simulink model "MODELODETURBINADERIOV9"  (R2018a)
settings: Solver=VariableStepAuto  StartTime=0.0  StopTime=0.5  FixedStep=50e-3  MaxStep=1e-4  RelTol=1e-3
undefined symbols (not defined in the file): A, B, beta, Ccc, Cinv, Dcc, den, Fr, J, K1Vo, K2Vo, Kb, Kp, Lcc, Linv, Lr, r, Rcc, Ri, Rinv, Rr, sigbuilder_block, T_d, Tc
libraries: powerlib x43, simulink x3, powerlib_meascontrol x1
settings Model: Creator=zni.uao  LastModifiedBy=cmparedes
settings SolverCC: ZeroCrossAlgorithm=Adaptive
settings OptimizationCC: LifeSpan=inf
settings DebuggingCC: SFExecutionAtInitializationDiag=none
settings HardwareCC: ProdBitPerPointer=32  ProdBitPerSizeT=32  ProdBitPerPtrDiffT=32  ProdLargestAtomicFloat=None  ProdWordSize=32  ProdHWDeviceType=Custom Processor->Custom
settings CodeAppCC: StateflowObjectComments=on
settings SimscapeCC: SimscapeNormalizeSystem=off

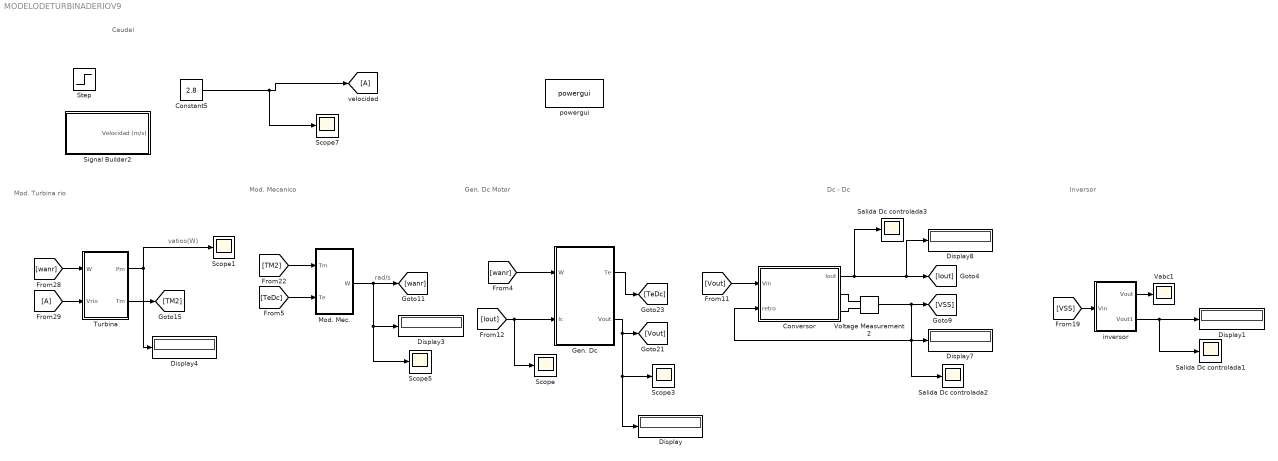
== system MODELODETURBINADERIOV9 ==
  note: rad/s
  note: Mod. Turbina rio
  note: Mod. Mecanico
  note: Caudal
  note: Gen. Dc Motor
  note: Dc - Dc
  note: Inversor
  note: vatios(W)
  Constant5 : Constant  Value=2.8
  Conversor : Subsystem
  Display{,1,3..4,7..8} (6 alike) : Display
  Gen. Dc : Subsystem
  Mod. Mec. : Subsystem
  Salida Dc controlada1 : Scope
  Salida Dc controlada2 : Scope
  Salida Dc controlada3 : Scope
  Scope{,1,3,5,7} (5 alike) : Scope
  Signal Builder2 : Subsystem  Tag=STV Subsys  LoadFcn=sigbuilder_block('load');  StartFcn=sigbuilder_block('start');  StopFcn=sigbuilder_block('stop');  ClipboardFcn=sigbuilder_block('clipboard');  mask(Sigbuilder block){tuvar=[0:10]}
      mask help: Simulink:masks:SigbuilderBlock_MD
      mask init:
      | if ~strcmp(get_param(bdroot(gcbh),'SimulationStatus'),'stopped') tuvar = sigbuilder_block('maskInit'); end
      settings: CopyFcn=sigbuilder_block('copy');  DeleteFcn=sigbuilder_block('delete');  ModelCloseFcn=sigbuilder_block('modelClose');  PreSaveFcn=sigbuilder_block('preSave');  PauseFcn=sigbuilder_block('pause');  ContinueFcn=sigbuilder_block('continue');  NameChangeFcn=sigbuilder_block('namechange');  OpenFcn=sigbuilder_block('open',[197.25 66 550.5 359.25 ]);  CloseFcn=sigbuilder_block('close');
      mask Display: plot(0, 0, 100, 100,[2, 2, 32, 32, 2], [68, 8, 8, 68, 68],[32, 2], [38, 38], [32, 19, 2],[53, 60, 44], [32, 17, 17, 2],[16, 16, 31, 31]);txt = getActiveGroup(gcbh);text(2, 100, txt,'verticalAlignment', 'top');
  Step : Step  Time=10  Before=2.5  After=2.888  SampleTime=0
  Turbina : Subsystem
  Vabc1 : Scope
  Voltage Measurement2 : powerlib/Measurements/Voltage Measurement  PhasorSimulation=off  OutputType=Complex  PSBequivalent=0
  inversor : Subsystem
  powergui : powerlib/powergui  Priority=1  SimulationMode=Continuous  SampleTime=50e-3  frequency=60  Iterations=50  frequencyindice=0  Pbase=100e6  ErrMax=1e-4  UnitsV=kV  UnitsW=MW  buscounter=0  FunctionMessages=off  echomessages=off  EnableUseOfTLC=off  CurrentSourceSwitches=off  DisableSnubberDevices=off  DisableRonSwitches=off  DisableVfSwitches=off  DisplayEquations=off  SolverType=Tustin/Backward Euler (TBE)  Interpol=off  ExternalGateDelay=off  methode=off  Ts=100  x0status=blocks  SPID=on  SwTol=0  HookPort=off  RestoreLinks=warning  ResistiveCurrentMeasurement=off  Frange=[0:2:500]  Ylog=off  Xlog=on  ShowGrid=off  save=off  variable=ZData  structure=0  ZoomFFT=off  StartTime=0.0  cycles=1  DisplayStyle=1  fundamental=60  FreqAxis=off  MaxFrequency=1000  frequencyindicesteady=0 Hz  RmsSteady=1  display=off
  wires:
  [wanr] -> Turbina/1(W)
  [A] -> Turbina/2(Vrio)
  Turbina/1(Pm) -> Scope1/1, Display4/1
  Turbina/2(Tm) -> [TM2]
  Mod. Mec./1(W) -> Display3/1, Scope5/1, [wanr]
  [TM2] -> Mod. Mec./1(Tm)
  Gen. Dc/1(Te) -> [TeDc]
  [TeDc] -> Mod. Mec./2(Te)
  Constant5/1 -> Scope7/1, [A]
  [wanr] -> Gen. Dc/1(W)
  [VSS] -> inversor/1(Vin)
  [Iout] -> Scope/1, Gen. Dc/2(Ic)
  Gen. Dc/2(Vout) -> [Vout], Scope3/1, Display/1
  Voltage Measurement2/1 -> [VSS], Conversor/2(retro), Salida Dc controlada2/1, Display7/1
  Conversor/1(Iout) -> Salida Dc controlada3/1, Display8/1, [Iout]
  inversor/1(Vout) -> Vabc1/1
  [Vout] -> Conversor/1(Vin)
  inversor/2(Vout1) -> Salida Dc controlada1/1, Display1/1
  connections:
  Voltage Measurement2/LConn1 -- Conversor/RConn1
  Voltage Measurement2/LConn2 -- Conversor/RConn2

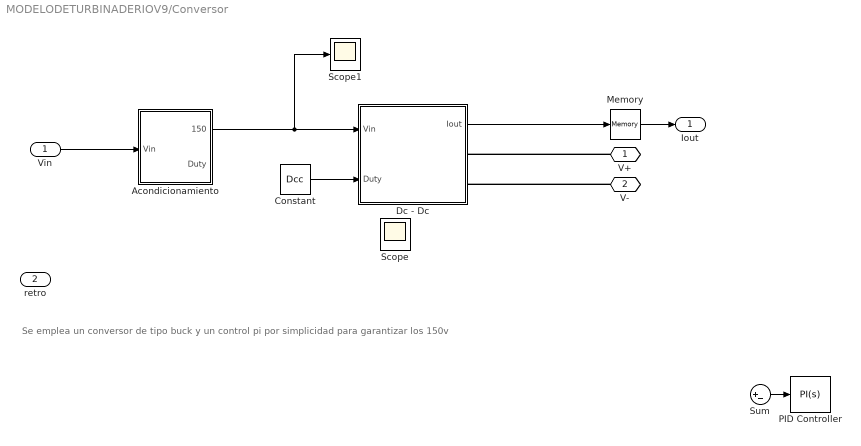
== system MODELODETURBINADERIOV9/Conversor ==
  note: Se emplea un conversor de tipo buck y un control pi por simplicidad para garantizar los 150v
  Vin : Inport
  retro : Inport  Port=2
  Acondicionamiento : Subsystem
  Constant : Constant  Value=Dcc
  Dc - Dc : Subsystem
  Memory : Memory
  PID Controller : simulink/Continuous/PID Controller  Controller=PI  TimeDomain=Continuous-time  SampleTime=-1  IntegratorMethod=Forward Euler  FilterMethod=Forward Euler  Form=Parallel  UseFilter=on  ControllerParametersSource=internal  P=0  I=49.9781304897077  D=1.18866706411967e-05  N=181963.738974805  InitialConditionSource=internal  InitialConditionForIntegrator=0  InitialConditionForFilter=0  ExternalReset=none  LimitOutput=off  UpperSaturationLimit=inf  LowerSaturationLimit=-inf  LinearizeAsGain=on  AntiWindupMode=none  Kb=1  TrackingMode=off  Kt=1  PParamMin=[]  PParamMax=[]  IParamMin=[]  IParamMax=[]  DParamMin=[]  DParamMax=[]  NParamMin=[]  NParamMax=[]  KbParamMin=[]  KbParamMax=[]  KtParamMin=[]  KtParamMax=[]  POutMin=[]  POutMax=[]  IOutMin=[]  IOutMax=[]  DOutMin=[]  DOutMax=[]  NOutMin=[]  NOutMax=[]  KbOutMin=[]  KbOutMax=[]  KtOutMin=[]  KtOutMax=[]  IntegratorOutMin=[]  IntegratorOutMax=[]  FilterOutMin=[]  FilterOutMax=[]  SumOutMin=[]  SumOutMax=[]  SumI1OutMin=[]  SumI1OutMax=[]  SumI2OutMin=[]  SumI2OutMax=[]  SumI3OutMin=[]  SumI3OutMax=[]  SumDOutMin=[]  SumDOutMax=[]  SaturationOutMin=[]  SaturationOutMax=[]  IntegratorContinuousStateAttributes=''  IntegratorStateMustResolveToSignalObject=off  IntegratorRTWStateStorageClass=Auto  FilterContinuousStateAttributes=''  FilterStateMustResolveToSignalObject=off  FilterRTWStateStorageClass=Auto  DifferentiatorICPrevScaledInput=0  DifferentiatorOutMin=[]  DifferentiatorOutMax=[]  InitialConditionSetting=State (most efficient)  FilterDiffOutCoefMin=[]  FilterDiffOutCoefMax=[]  SumDenOutMin=[]  SumDenOutMax=[]  SumNumOutMin=[]  SumNumOutMax=[]  ReciprocalOutMin=[]  ReciprocalOutMax=[]  DivideOutMin=[]  DivideOutMax=[]  TunerSelectOption=Transfer Function Based (PID Tuner App)
  Scope : Scope
  Scope1 : Scope
  Sum : Sum  Inputs=|+-
  V+ : PMIOPort  Side=Right
  V- : PMIOPort  Port=2  Side=Right
  Iout : Outport
  wires:
  Dc - Dc/1(Iout) -> Memory/1
  Acondicionamiento/1(150) -> Scope1/1, Dc - Dc/1(Vin)
  Memory/1 -> Iout/1
  Vin/1 -> Acondicionamiento/1(Vin)
  ? -> Sum/1
  Sum/1 -> PID Controller/1
  ? -> Sum/2
  Constant/1 -> Dc - Dc/2(Duty)
  connections:
  V+/RConn1 -- Dc - Dc/RConn1
  V-/RConn1 -- Dc - Dc/RConn2

== system MODELODETURBINADERIOV9/Gen. Dc ==
  note: Calculo del par electrico con la corriente en la carga
  note: Se emplean parametro de un motor dc para 18.5Kw debido a que fueron con los que mejor trabajo
  W : Inport
  Ic : Inport  Port=2
  Motor iman. : Subsystem
  Par elec. : Subsystem
  Te : Outport
  Vout : Outport  Port=2
  wires:
  Motor iman./1(Out1) -> Vout/1
  Par elec./1(Te) -> Te/1
  W/1 -> Motor iman./2(W)
  Ic/1 -> Par elec./1(Ic), Motor iman./1(I)

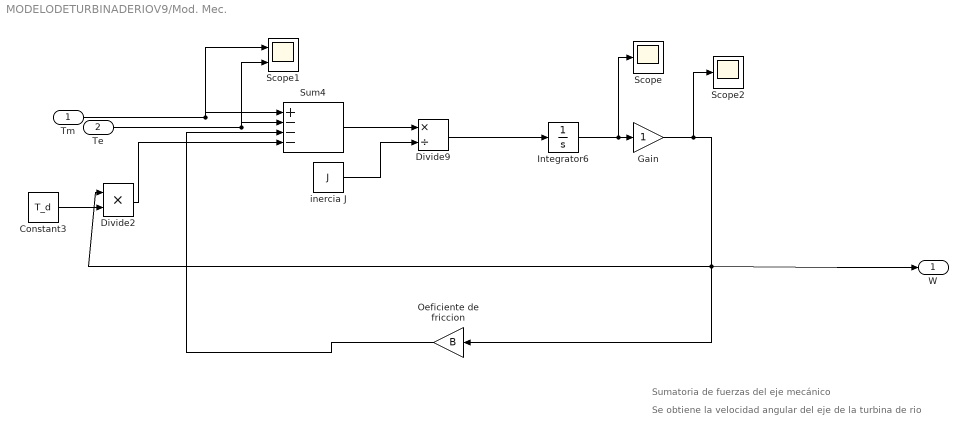
== system MODELODETURBINADERIOV9/Mod. Mec. ==
  note: Se obtiene la velocidad angular del eje de la turbina de rio
  note: Sumatoria de fuerzas del eje mecánico
  Tm : Inport
  Te : Inport  Port=2
  Constant3 : Constant  Value=T_d
  Divide2 : Product  Inputs=**
  Divide9 : Product  Inputs=*/
  Gain : Gain
  Integrator6 : Integrator  InitialCondition=10
  Oeficiente de friccion : Gain  Gain=B
  Scope : Scope
  Scope1 : Scope  NumInputPorts=2
  Scope2 : Scope
  Sum4 : Sum  Inputs=|+---
  inercia J : Constant  Value=J
  W : Outport
  wires:
  inercia J/1 -> Divide9/2
  Constant3/1 -> Divide2/2
  Divide2/1 -> Sum4/4
  Oeficiente de friccion/1 -> Sum4/3
  Sum4/1 -> Divide9/1
  Tm/1 -> Scope1/1, Sum4/1
  Te/1 -> Scope1/2, Sum4/2
  Divide9/1 -> Integrator6/1
  Integrator6/1 -> Scope/1, Gain/1
  Gain/1 -> Scope2/1, Oeficiente de friccion/1, W/1, Divide2/1

== system MODELODETURBINADERIOV9/Signal Builder2 ==
  Demux : Demux  Tag=STV Demux  Outputs=1
  FromWs : FromWorkspace  Tag=STV FromWs  VariableName=tuvar  SampleTime=0
      SigBuilderData=|
      | common.afterFinalStr = 'Extrapolate'
      | common.sampleTime = 0
      | dataSet.timeRange = [0 0.1]
      | dataSet.name = 'Group 1'
      | sbobj.Groups.Name = 'Group 1'
      | sbobj.Groups.Signals.Name = 'Velocidad (m/s)'
      | sbobj.Groups.Signals.XData = [0 0.01 0.01 0.02 0.02 0.0298 0.0298 0.0398 0.0498 0.06 0.1]
      | sbobj.Groups.Signals.YData = [2 2 2.5 2.5 2.595 2.595 2.8 2.8 2.8 2.8 2.8]
      | sbobj.Groups.TimeRange = [0 0.1]
  Velocidad (m/s) : Outport  Tag=STV Outport
  wires:
  FromWs/1 -> Demux/1
  Demux/1 -> Velocidad (m/s)/1

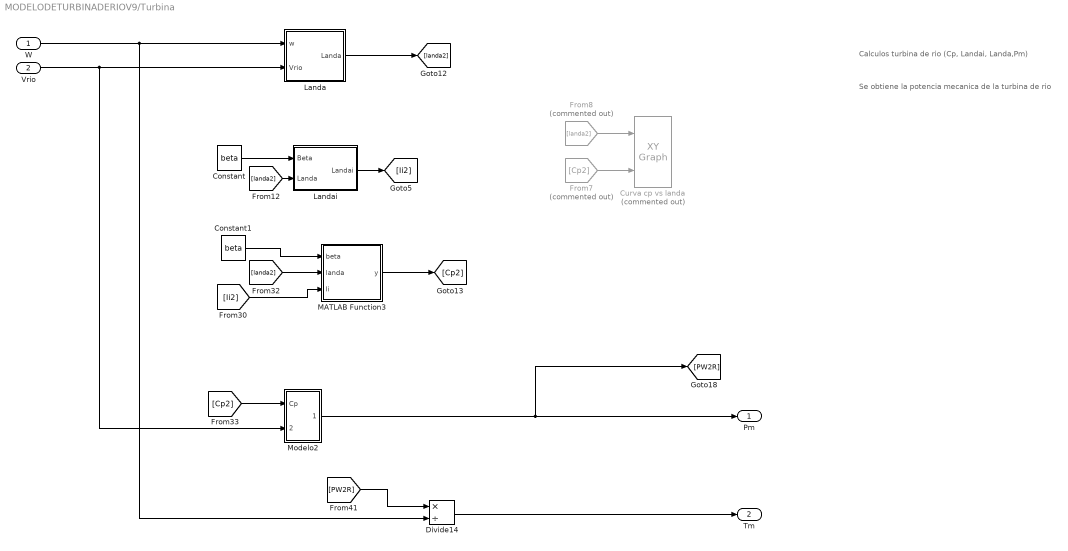
== system MODELODETURBINADERIOV9/Turbina ==
  note: Calculos turbina de rio (Cp, Landai, Landa,Pm)
  note: Se obtiene la potencia mecanica de la turbina de rio
  W : Inport
  Vrio : Inport  Port=2
  Constant : Constant  Value=beta
  Constant1 : Constant  Value=beta
  Curva cp vs landa : simulink/Sinks/XY Graph  Commented=on  xmin=1  xmax=20  ymin=0  ymax=0.56  st=0.1
  Divide14 : Product  Inputs=*/
  From7 : From  Commented=on  GotoTag=Cp2
  From8 : From  Commented=on  GotoTag=landa2
  Landa : Subsystem
  Landai : Subsystem
  MATLAB Function3 : MATLAB Function  TreatAsAtomicUnit=on
  Modelo2 : Subsystem
  Pm : Outport
  Tm : Outport  Port=2
  wires:
  Constant1/1 -> MATLAB Function3/1(beta)
  Divide14/1 -> Tm/1
  [Ii2] -> MATLAB Function3/3(Ii)
  [Cp2] -> Modelo2/1(Cp)
  [PW2R] -> Divide14/1
  W/1 -> Divide14/2, Landa/1(w)
  [landa2] -> MATLAB Function3/2(landa)
  Vrio/1 -> Modelo2/2(Vrio), Landa/2(Vrio)
  Landa/1(Landa) -> [landa2]
  MATLAB Function3/1(y) -> [Cp2]
  From8/1 -> Curva cp vs landa/1
  Constant/1 -> Landai/1(Beta)
  [landa2] -> Landai/2(Landa)
  Modelo2/1(Pm) -> [PW2R], Pm/1
  Landai/1(Landai) -> [Ii2]
  From7/1 -> Curva cp vs landa/2

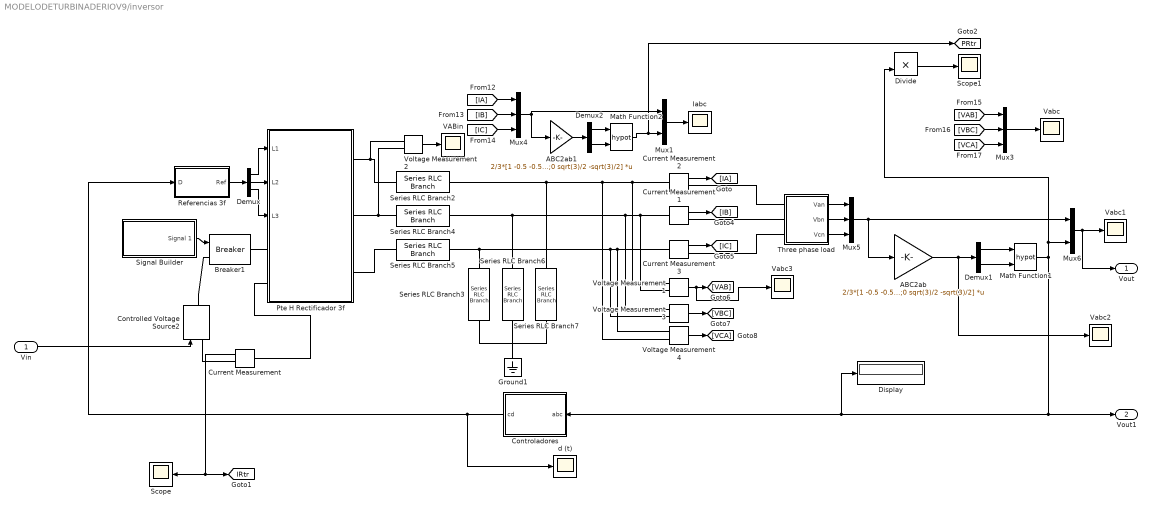
== system MODELODETURBINADERIOV9/inversor ==
  Vin : Inport
  ABC2ab : Gain  Gain=2/3*[1 -0.5 -0.5;0 sqrt(3)/2 -sqrt(3)/2]  Multiplication=Matrix(K*u)  SaturateOnIntegerOverflow=on  OutDataTypeStr=Inherit: Same as input  ParamDataTypeStr=Inherit: Same as input
  ABC2ab1 : Gain  Gain=2/3*[1 -0.5 -0.5;0 sqrt(3)/2 -sqrt(3)/2]  Multiplication=Matrix(K*u)  SaturateOnIntegerOverflow=on  OutDataTypeStr=Inherit: Same as input  ParamDataTypeStr=Inherit: Same as input
  Breaker1 : powerlib/Elements/Breaker  InitialState=0  SwitchingTimes="[ 1/60  5/60 ]"  External=on  BreakerResistance=0.01  SnubberResistance=1e6  SnubberCapacitance=inf  Measurements=None  MoreParameters=off  NoBreakLoop=off
      settings: SourceProductName=Simscape Power Systems
  Controladores : Subsystem
  Controlled Voltage Source2 : powerlib/Electrical Sources/Controlled Voltage Source  Initialize=on  Source_Type=DC  Amplitude=150  Phase=0  Frequency=0  Measurements=None
  Current Measurement{,1..3} (4 alike) : powerlib/Measurements/Current Measurement  PhasorSimulation=off  OutputType=Complex  PSBequivalent=0
  Demux : Demux  Outputs=3
  Demux1 : Demux  Outputs=2
  Demux2 : Demux  Outputs=2
  Display : Display
  Divide : Product  Inputs=**
  Ground1 : powerlib/Elements/Ground  LConnTagsString=a
  Iabc : Scope
  Math Function1 : Math  Operator=hypot  SaturateOnIntegerOverflow=on
  Math Function2 : Math  Operator=hypot  SaturateOnIntegerOverflow=on
  Mux1 : Mux  Inputs=2
  Mux3 : Mux  Inputs=3
  Mux4 : Mux  Inputs=3
  Mux5 : Mux  Inputs=3
  Mux6 : Mux  Inputs=2
  Pte H Rectificador 3f : Subsystem
  Referencias 3f : Subsystem
  Scope : Scope
  Scope1 : Scope
  Series RLC Branch2 : powerlib/Elements/Series RLC Branch  LConnTagsString=__new0  RConnTagsString=__new0  BranchType=RL  Resistance=Rinv  Inductance=Linv  SetiL0=off  InitialCurrent=0  Capacitance=1.0  Setx0=off  InitialVoltage=0  Measurements=None
  Series RLC Branch3 : powerlib/Elements/Series RLC Branch  LConnTagsString=__new0  RConnTagsString=__new0  BranchType=C  Resistance=0.01  Inductance=1e-3  SetiL0=off  InitialCurrent=0  Capacitance=Cinv  Setx0=on  InitialVoltage=311  Measurements=None
  Series RLC Branch4 : powerlib/Elements/Series RLC Branch  LConnTagsString=__new0  RConnTagsString=__new0  BranchType=RL  Resistance=Rinv  Inductance=Linv  SetiL0=off  InitialCurrent=0  Capacitance=1.0  Setx0=off  InitialVoltage=0  Measurements=None
  Series RLC Branch5 : powerlib/Elements/Series RLC Branch  LConnTagsString=__new0  RConnTagsString=__new0  BranchType=RL  Resistance=Rinv  Inductance=Linv  SetiL0=off  InitialCurrent=0  Capacitance=1.0  Setx0=off  InitialVoltage=0  Measurements=None
  Series RLC Branch6 : powerlib/Elements/Series RLC Branch  LConnTagsString=__new0  RConnTagsString=__new0  BranchType=C  Resistance=0.01  Inductance=1e-3  SetiL0=off  InitialCurrent=0  Capacitance=Cinv  Setx0=on  InitialVoltage=311  Measurements=None
  Series RLC Branch7 : powerlib/Elements/Series RLC Branch  LConnTagsString=__new0  RConnTagsString=__new0  BranchType=C  Resistance=0.01  Inductance=1e-3  SetiL0=off  InitialCurrent=0  Capacitance=Cinv  Setx0=on  InitialVoltage=311  Measurements=None
  Signal Builder : Subsystem  Tag=STV Subsys  LoadFcn=sigbuilder_block('load');  StartFcn=sigbuilder_block('start');  StopFcn=sigbuilder_block('stop');  ClipboardFcn=sigbuilder_block('clipboard');  mask(Sigbuilder block){tuvar=[0:10]}
      mask help: Sigbuilder GUI
      mask init:
      | if ~strcmp(get_param(bdroot(gcbh),'SimulationStatus'),'stopped') tuvar = sigbuilder_block('maskInit'); end
      settings: CopyFcn=sigbuilder_block('copy');  DeleteFcn=sigbuilder_block('delete');  ModelCloseFcn=sigbuilder_block('modelClose');  PreSaveFcn=sigbuilder_block('preSave');  PauseFcn=sigbuilder_block('pause')  ContinueFcn=sigbuilder_block('continue')  NameChangeFcn=sigbuilder_block('namechange');  OpenFcn=sigbuilder_block('open',[437.25 117 550.5 399 ]);  CloseFcn=sigbuilder_block('close');
      mask Display: plot(0, 0, 100, 100,[2, 2, 32, 32, 2], [68, 8, 8, 68, 68],[32, 2], [38, 38], [32, 19, 2],[53, 60, 44], [32, 17, 17, 2],[16, 16, 31, 31]);txt = getActiveGroup(gcbh);text(2, 100, txt,'verticalAlignment', 'top');
  Three phase load : Subsystem
  VABin : Scope
  Vabc{,1..3} (4 alike) : Scope
  Voltage Measurement{1..4} (4 alike) : powerlib/Measurements/Voltage Measurement  PhasorSimulation=off  OutputType=Complex  PSBequivalent=0
  d (t) : Scope
  Vout : Outport
  Vout1 : Outport  Port=2
  tag scope: IRtr=global, PRtr=global
  wires:
  Demux/3 -> Pte H Rectificador 3f/3(L3)
  Referencias 3f/1(Ref) -> Demux/1
  [VBC] -> Mux3/2
  Three phase load/3(Vcn) -> Mux5/3
  Three phase load/1(Van) -> Mux5/1
  ABC2ab1/1 -> Demux2/1
  Current Measurement3/1 -> [IC]
  Mux5/1 -> Mux6/1, ABC2ab/1
  Demux2/1 -> Math Function2/1
  [VCA] -> Mux3/3
  [IA] -> Mux4/1
  Three phase load/2(Vbn) -> Mux5/2
  Voltage Measurement4/1 -> [VCA]
  Mux3/1 -> Vabc/1
  Demux2/2 -> Math Function2/2
  [VAB] -> Mux3/1
  Current Measurement2/1 -> [IA]
  Demux1/2 -> Math Function1/2
  Mux1/1 -> Iabc/1
  Current Measurement1/1 -> [IB]
  Voltage Measurement1/1 -> Vabc3/1, [VAB]
  Controladores/1(cd) -> d (t)/1, Referencias 3f/1(D)
  Math Function2/1 -> [PRtr], Mux1/2
  Voltage Measurement3/1 -> [VBC]
  ABC2ab/1 -> Demux1/1, Vabc2/1
  Demux/1 -> Pte H Rectificador 3f/1(L1)
  Math Function1/1 -> Divide/2, Mux6/2, Vout1/1, Controladores/1(abc), Display/1
  Demux/2 -> Pte H Rectificador 3f/2(L2)
  Mux4/1 -> ABC2ab1/1, Mux1/1
  [IB] -> Mux4/2
  Mux6/1 -> Vout/1, Vabc1/1
  Demux1/1 -> Math Function1/1
  [IC] -> Mux4/3
  Vin/1 -> Controlled Voltage Source2/1
  Signal Builder/1(Signal 1) -> Breaker1/1
  Voltage Measurement2/1 -> VABin/1
  Current Measurement/1 -> [IRtr], Scope/1
  Divide/1 -> Scope1/1
  connections:
  Three phase load/LConn1 -- Current Measurement2/RConn1
  Series RLC Branch5/LConn1 -- Pte H Rectificador 3f/RConn3
  Series RLC Branch3/RConn1 -- Ground1/LConn1
  Series RLC Branch6/LConn1 -- Voltage Measurement1/LConn2 -- Current Measurement1/LConn1 -- Voltage Measurement3/LConn1 -- Series RLC Branch4/RConn1
  Series RLC Branch3/LConn1 -- Current Measurement3/LConn1 -- Voltage Measurement4/LConn1 -- Voltage Measurement3/LConn2 -- Series RLC Branch5/RConn1
  Series RLC Branch7/RConn1 -- Series RLC Branch6/RConn1
  Three phase load/LConn3 -- Current Measurement3/RConn1
  Series RLC Branch4/LConn1 -- Voltage Measurement2/LConn2 -- Pte H Rectificador 3f/RConn2
  Three phase load/LConn2 -- Current Measurement1/RConn1
  Series RLC Branch2/RConn1 -- Series RLC Branch7/LConn1 -- Voltage Measurement1/LConn1 -- Current Measurement2/LConn1 -- Voltage Measurement4/LConn2
  Series RLC Branch2/LConn1 -- Voltage Measurement2/LConn1 -- Pte H Rectificador 3f/RConn1
  Controlled Voltage Source2/RConn1 -- Breaker1/LConn1
  Breaker1/RConn1 -- Pte H Rectificador 3f/LConn1
  Current Measurement/RConn1 -- Controlled Voltage Source2/LConn1
  Current Measurement/LConn1 -- Pte H Rectificador 3f/LConn2

== system MODELODETURBINADERIOV9/Conversor/Acondicionamiento ==
  note: Se garantiza una entrada fija a 150, pero si la tension de entrada desciende
      | se deja su valor original y se calcula con ello el ciclo Duty
  Vin : Inport
  Constant1 : Constant  Value=150
  Divide : Product  Inputs=**
  Divide1 : Product  Inputs=*/
  Saturation : Saturate  UpperLimit=1  LowerLimit=0
  150 : Outport
  Duty : Outport  Port=2
  wires:
  Divide1/1 -> Saturation/1
  Divide/1 -> 150/1
  Saturation/1 -> Duty/1, Divide/2
  Constant1/1 -> Divide1/1
  Vin/1 -> Divide/1, Divide1/2

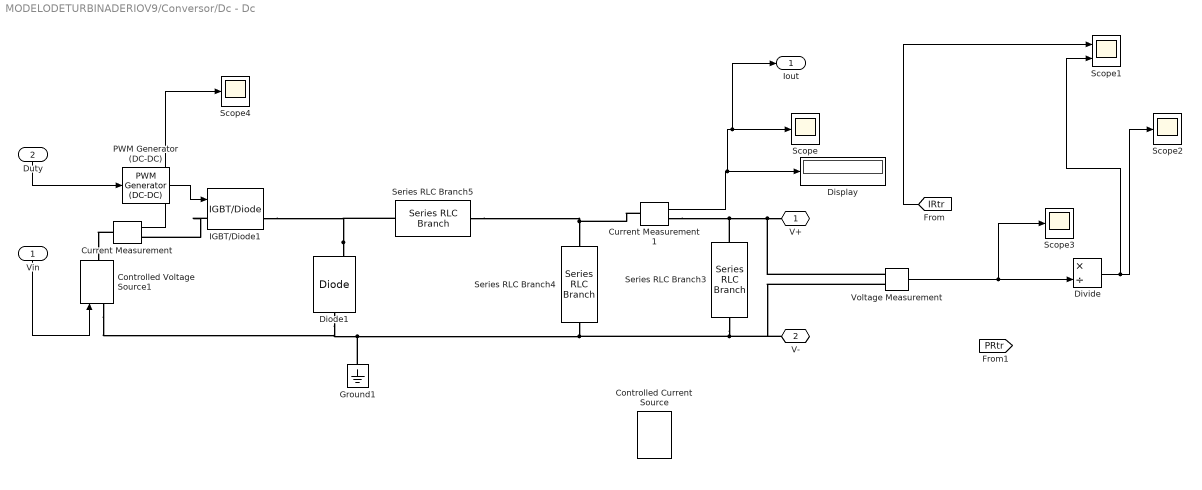
== system MODELODETURBINADERIOV9/Conversor/Dc - Dc ==
  Vin : Inport
  Duty : Inport  Port=2
  Controlled Current Source : powerlib/Electrical Sources/Controlled Current Source  Initialize=on  Source_Type=AC  Amplitude=0  Phase=0  Frequency=0  Measurements=None
  Controlled Voltage Source1 : powerlib/Electrical Sources/Controlled Voltage Source  Initialize=on  Source_Type=DC  Amplitude=0  Phase=0  Frequency=0  Measurements=None
  Current Measurement : powerlib/Measurements/Current Measurement  PhasorSimulation=off  OutputType=Complex  PSBequivalent=0
  Current Measurement1 : powerlib/Measurements/Current Measurement  PhasorSimulation=off  OutputType=Complex  PSBequivalent=0
  Diode1 : powerlib/Power Electronics/Diode  Ron=0.001  Lon=0  Vf=0.8  IC=0  UseSnubber=0  Rs=500  Cs=250e-9  Measurements=on
  Display : Display
  Divide : Product  Inputs=*/
  Ground1 : powerlib/Elements/Ground  LConnTagsString=a
  IGBT/Diode1 : powerlib/Power Electronics/IGBT//Diode  Ron=1e-3  Rs=1e5  Cs=inf  Measurements=on
  PWM Generator (DC-DC) : powerlib_meascontrol/Pulse & Signal Generators/PWM Generator (DC-DC)  Fsw=20000  Ts=0.000005
  Scope{,2..4} (4 alike) : Scope
  Scope1 : Scope  NumInputPorts=2
  Series RLC Branch3 : powerlib/Elements/Series RLC Branch  LConnTagsString=__new0  RConnTagsString=__new0  BranchType=R  Resistance=Rcc  Inductance=1e-3  SetiL0=off  InitialCurrent=0  Capacitance=1e-6  Setx0=off  InitialVoltage=0  Measurements=None
  Series RLC Branch4 : powerlib/Elements/Series RLC Branch  LConnTagsString=__new0  RConnTagsString=__new0  BranchType=C  Resistance=1  Inductance=1e-3  SetiL0=off  InitialCurrent=0  Capacitance=Ccc  Setx0=off  InitialVoltage=0  Measurements=None
  Series RLC Branch5 : powerlib/Elements/Series RLC Branch  LConnTagsString=__new0  RConnTagsString=__new0  BranchType=L  Resistance=1  Inductance=Lcc  SetiL0=off  InitialCurrent=0  Capacitance=1e-6  Setx0=off  InitialVoltage=0  Measurements=None
  Voltage Measurement : powerlib/Measurements/Voltage Measurement  PhasorSimulation=off  OutputType=Complex  PSBequivalent=0
  V+ : PMIOPort  Side=Right
  V- : PMIOPort  Port=2  Side=Right
  Iout : Outport
  wires:
  Duty/1 -> PWM Generator (DC-DC)/1
  PWM Generator (DC-DC)/1 -> IGBT/Diode1/1
  Vin/1 -> Controlled Voltage Source1/1
  Current Measurement1/1 -> Iout/1, Scope/1, Display/1
  Voltage Measurement/1 -> Scope3/1, Divide/2
  Divide/1 -> Scope1/2, Scope2/1
  [IRtr] -> Scope1/1
  Current Measurement/1 -> Scope4/1
  connections:
  Diode1/LConn1 -- Controlled Voltage Source1/LConn1 -- Ground1/LConn1 -- Series RLC Branch3/RConn1 -- Voltage Measurement/LConn2 -- V-/RConn1 -- Series RLC Branch4/RConn1
  Diode1/RConn1 -- IGBT/Diode1/RConn1 -- Series RLC Branch5/RConn1
  Series RLC Branch5/LConn1 -- Current Measurement1/LConn1 -- Series RLC Branch4/LConn1
  IGBT/Diode1/LConn1 -- Current Measurement/RConn1
  Current Measurement/LConn1 -- Controlled Voltage Source1/RConn1
  Current Measurement1/RConn1 -- Series RLC Branch3/LConn1 -- Voltage Measurement/LConn1 -- V+/RConn1

== system MODELODETURBINADERIOV9/Gen. Dc/Motor iman. ==
  note: Se obtiene la tension del generador a partir de una velocidad angular
  note: y una corriente retroalimentada del conversor dc-dc
  I : Inport
  W : Inport  Port=2
  Constant1 : Constant  Value=Kb
  Constant2 : Constant  Value=Ri
  Divide6 : Product  Inputs=**  SaturateOnIntegerOverflow=on  RndMeth=Zero
  Divide7 : Product  Inputs=**  SaturateOnIntegerOverflow=on  RndMeth=Zero
  Sum1 : Sum
  Out1 : Outport
  wires:
  Divide7/1 -> Sum1/2
  Divide6/1 -> Sum1/1
  I/1 -> Divide7/2
  Constant2/1 -> Divide7/1
  Constant1/1 -> Divide6/1
  W/1 -> Divide6/2
  Sum1/1 -> Out1/1

== system MODELODETURBINADERIOV9/Gen. Dc/Par elec. ==
  Ic : Inport
  Constant2 : Constant  Value=Kp
  Divide2 : Product  Inputs=**
  Te : Outport
  wires:
  Ic/1 -> Divide2/1
  Constant2/1 -> Divide2/2
  Divide2/1 -> Te/1

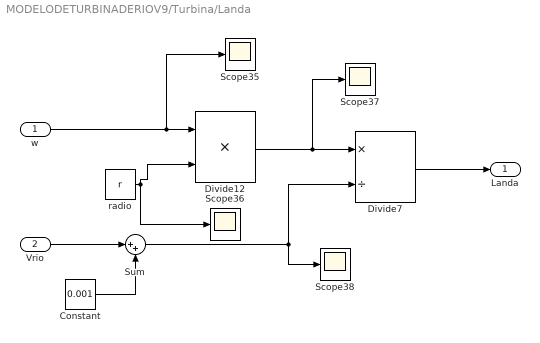
== system MODELODETURBINADERIOV9/Turbina/Landa ==
  w : Inport
  Vrio : Inport  Port=2
  Constant : Constant  Value=0.001
  Divide12 : Product  Inputs=**
  Divide7 : Product  Inputs=*/
  Scope{35..38} (4 alike) : Scope
  Sum : Sum  Inputs=|++
  radio : Constant  Value=r
  Landa : Outport
  wires:
  Divide7/1 -> Landa/1
  radio/1 -> Divide12/2, Scope36/1
  Divide12/1 -> Scope37/1, Divide7/1
  w/1 -> Scope35/1, Divide12/1
  Vrio/1 -> Sum/1
  Sum/1 -> Scope38/1, Divide7/2
  Constant/1 -> Sum/2

== system MODELODETURBINADERIOV9/Turbina/Landai ==
  Beta : Inport
  Landa : Inport  Port=2
  lamdai : MATLAB Function  TreatAsAtomicUnit=on
  Landai : Outport
  wires:
  lamdai/1(Ii) -> Landai/1
  Landa/1 -> lamdai/2(landa)
  Beta/1 -> lamdai/1(beta)

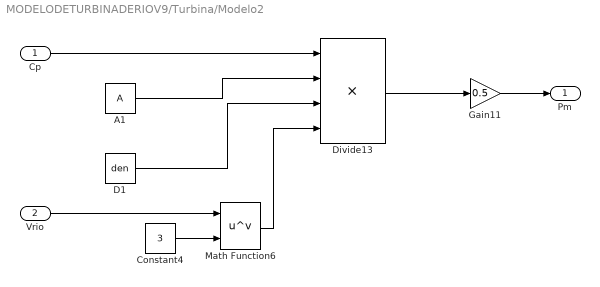
== system MODELODETURBINADERIOV9/Turbina/Modelo2 ==
  Cp : Inport
  Vrio : Inport  Port=2
  A1 : Constant  Value=A
  Constant4 : Constant  Value=3
  D1 : Constant  Value=den
  Divide13 : Product  Inputs=****  SaturateOnIntegerOverflow=on  RndMeth=Zero
  Gain11 : Gain  Gain=0.5
  Math Function6 : Math  Operator=pow  SaturateOnIntegerOverflow=on
  Pm : Outport
  wires:
  Constant4/1 -> Math Function6/2
  Divide13/1 -> Gain11/1
  D1/1 -> Divide13/3
  Cp/1 -> Divide13/1
  Gain11/1 -> Pm/1
  A1/1 -> Divide13/2
  Vrio/1 -> Math Function6/1
  Math Function6/1 -> Divide13/4

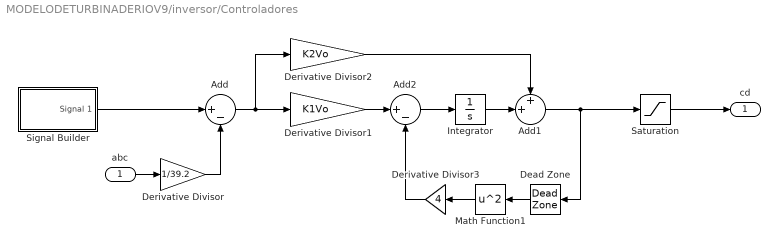
== system MODELODETURBINADERIOV9/inversor/Controladores ==
  abc : Inport
  Add : Sum  Inputs=|+-
  Add1 : Sum  Inputs=++|
  Add2 : Sum  Inputs=|+-
  Dead Zone : DeadZone  LowerValue=-1  UpperValue=1  SaturateOnIntegerOverflow=on
  Derivative Divisor : Gain  Gain=1/39.2  SaturateOnIntegerOverflow=on  OutDataTypeStr=Inherit: Same as input  ParamDataTypeStr=Inherit: Same as input
  Derivative Divisor1 : Gain  Gain=K1Vo  SaturateOnIntegerOverflow=on  OutDataTypeStr=Inherit: Same as input  ParamDataTypeStr=Inherit: Same as input
  Derivative Divisor2 : Gain  Gain=K2Vo  SaturateOnIntegerOverflow=on  OutDataTypeStr=Inherit: Same as input  ParamDataTypeStr=Inherit: Same as input
  Derivative Divisor3 : Gain  Gain=4  SaturateOnIntegerOverflow=on  OutDataTypeStr=Inherit: Same as input  ParamDataTypeStr=Inherit: Same as input
  Integrator : Integrator
  Math Function1 : Math  Operator=square  SaturateOnIntegerOverflow=on
  Saturation : Saturate  UpperLimit=1  LowerLimit=-1
  Signal Builder : Subsystem  Tag=STV Subsys  LoadFcn=sigbuilder_block('load');  StartFcn=sigbuilder_block('start');  StopFcn=sigbuilder_block('stop');  ClipboardFcn=sigbuilder_block('clipboard');  mask(Sigbuilder block){tuvar=[0:10]}
      mask help: Sigbuilder GUI
      mask init:
      | if ~strcmp(get_param(bdroot(gcbh),'SimulationStatus'),'stopped') tuvar = sigbuilder_block('maskInit'); end
      settings: CopyFcn=sigbuilder_block('copy');  DeleteFcn=sigbuilder_block('delete');  ModelCloseFcn=sigbuilder_block('modelClose');  PreSaveFcn=sigbuilder_block('preSave');  PauseFcn=sigbuilder_block('pause')  ContinueFcn=sigbuilder_block('continue')  NameChangeFcn=sigbuilder_block('namechange');  OpenFcn=sigbuilder_block('open',[6 24 765 492 ]);  CloseFcn=sigbuilder_block('close');
      mask Display: plot(0, 0, 100, 100,[2, 2, 32, 32, 2], [68, 8, 8, 68, 68],[32, 2], [38, 38], [32, 19, 2],[53, 60, 44], [32, 17, 17, 2],[16, 16, 31, 31]);txt = getActiveGroup(gcbh);text(2, 100, txt,'verticalAlignment', 'top');
  cd : Outport
  wires:
  Signal Builder/1(Signal 1) -> Add/1
  abc/1 -> Derivative Divisor/1
  Derivative Divisor/1 -> Add/2
  Add/1 -> Derivative Divisor1/1, Derivative Divisor2/1
  Integrator/1 -> Add1/2
  Derivative Divisor2/1 -> Add1/1
  Add1/1 -> Saturation/1, Dead Zone/1
  Saturation/1 -> cd/1
  Add2/1 -> Integrator/1
  Derivative Divisor1/1 -> Add2/1
  Dead Zone/1 -> Math Function1/1
  Derivative Divisor3/1 -> Add2/2
  Math Function1/1 -> Derivative Divisor3/1

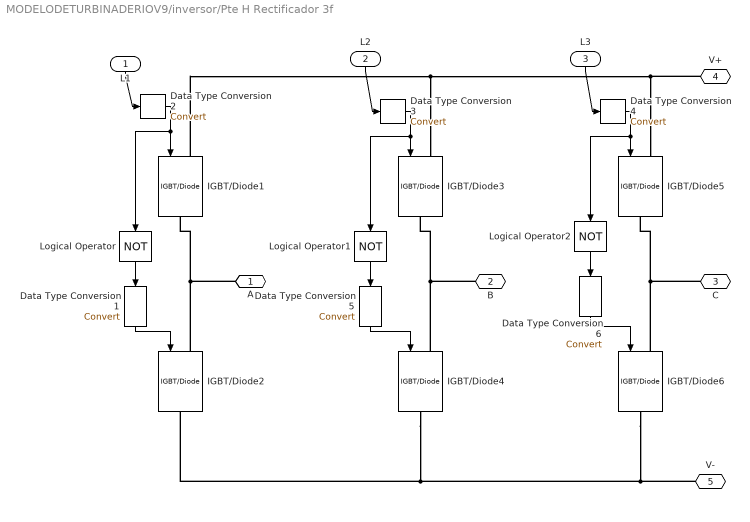
== system MODELODETURBINADERIOV9/inversor/Pte H Rectificador 3f ==
  L1 : Inport
  L2 : Inport  Port=2
  L3 : Inport  Port=3
  Data Type Conversion{1..6} (6 alike) : DataTypeConversion
  IGBT/Diode{1..6} (6 alike) : powerlib/Power Electronics/IGBT//Diode  Ron=1e-3  Rs=1e5  Cs=inf  Measurements=off
  Logical Operator : Logic  Operator=NOT  AllPortsSameDT=off  OutDataTypeStr=boolean
  Logical Operator1 : Logic  Operator=NOT  AllPortsSameDT=off  OutDataTypeStr=boolean
  Logical Operator2 : Logic  Operator=NOT  AllPortsSameDT=off  OutDataTypeStr=boolean
  A : PMIOPort  Side=Right
  B : PMIOPort  Port=2  Side=Right
  C : PMIOPort  Port=3  Side=Right
  V+ : PMIOPort  Port=4  Side=Left
  V- : PMIOPort  Port=5  Side=Left
  wires:
  L1/1 -> Data Type Conversion2/1
  L2/1 -> Data Type Conversion3/1
  L3/1 -> Data Type Conversion4/1
  Logical Operator/1 -> Data Type Conversion1/1
  Data Type Conversion2/1 -> IGBT/Diode1/1, Logical Operator/1
  Data Type Conversion3/1 -> IGBT/Diode3/1, Logical Operator1/1
  Data Type Conversion4/1 -> IGBT/Diode5/1, Logical Operator2/1
  Logical Operator1/1 -> Data Type Conversion5/1
  Logical Operator2/1 -> Data Type Conversion6/1
  Data Type Conversion1/1 -> IGBT/Diode2/1
  Data Type Conversion5/1 -> IGBT/Diode4/1
  Data Type Conversion6/1 -> IGBT/Diode6/1
  connections:
  IGBT/Diode2/LConn1 -- IGBT/Diode1/RConn1 -- A/RConn1
  IGBT/Diode4/LConn1 -- IGBT/Diode3/RConn1 -- B/RConn1
  IGBT/Diode6/RConn1 -- IGBT/Diode2/RConn1 -- IGBT/Diode4/RConn1 -- V-/RConn1
  IGBT/Diode1/LConn1 -- IGBT/Diode3/LConn1 -- IGBT/Diode5/LConn1 -- V+/RConn1
  IGBT/Diode6/LConn1 -- IGBT/Diode5/RConn1 -- C/RConn1

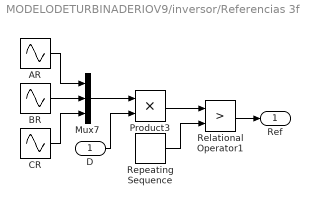
== system MODELODETURBINADERIOV9/inversor/Referencias 3f ==
  D : Inport
  AR : Sin  Frequency=Fr*2*pi  SampleTime=0
  BR : Sin  Frequency=Fr*2*pi  Phase=-2*pi/3  SampleTime=0
  CR : Sin  Frequency=Fr*2*pi  Phase=2*pi/3  SampleTime=0
  Mux7 : Mux  Inputs=3
  Product3 : Product  OutDataTypeStr=double  RndMeth=Zero
  Relational Operator1 : RelationalOperator  Operator=>  OutDataTypeStr=boolean  RndMeth=Nearest
  Repeating Sequence : simulink/Sources/Repeating Sequence  rep_seq_t=[0 Tc/2 Tc]  rep_seq_y=[-1 1 -1]
  Ref : Outport
  wires:
  CR/1 -> Mux7/3
  BR/1 -> Mux7/2
  AR/1 -> Mux7/1
  Product3/1 -> Relational Operator1/1
  Repeating Sequence/1 -> Relational Operator1/2
  Mux7/1 -> Product3/1
  D/1 -> Product3/2
  Relational Operator1/1 -> Ref/1

== system MODELODETURBINADERIOV9/inversor/Signal Builder ==
  Demux : Demux  Tag=STV Demux  Outputs=1
  FromWs : FromWorkspace  Tag=STV FromWs  VariableName=tuvar  SampleTime=0
      SigBuilderData=|
      | common.afterFinalStr = 'Extrapolate'
      | common.sampleTime = 0
      | dataSet.timeRange = [0 0.5]
      | dataSet.name = 'Group 1'
      | sbobj.Name = 'Signal Builder'
      | sbobj.Groups.Name = 'Group 1'
      | sbobj.Groups.Signals.Name = 'Signal 1'
      | sbobj.Groups.Signals.XData = [0 0.1 0.1 0.5]
      | sbobj.Groups.Signals.YData = [0 0 1 1]
      | sbobj.Groups.TimeRange = [0 0.5]
  Signal 1 : Outport  Tag=STV Outport
  wires:
  Demux/1 -> Signal 1/1
  FromWs/1 -> Demux/1

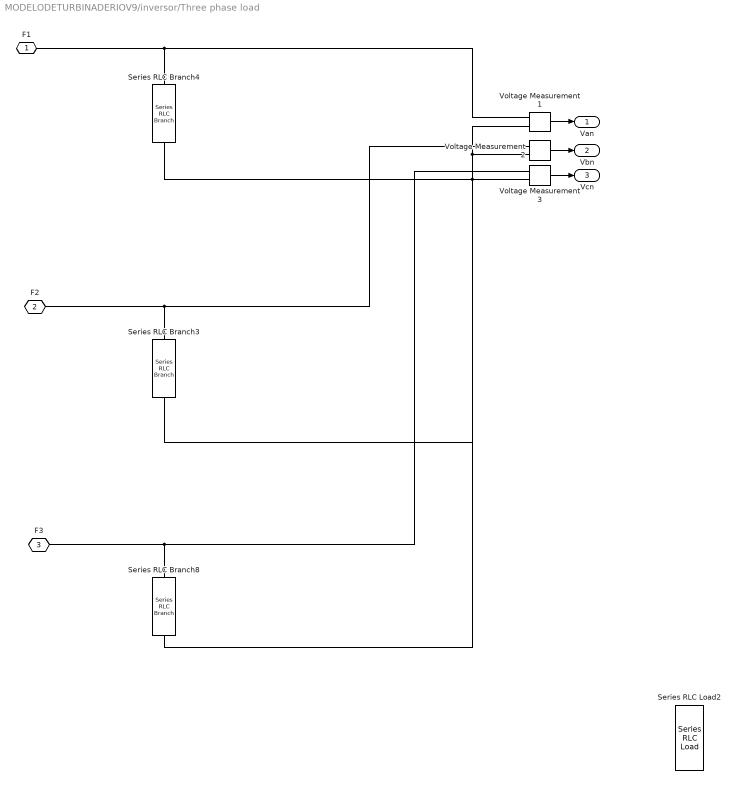
== system MODELODETURBINADERIOV9/inversor/Three phase load ==
  Series RLC Branch3 : powerlib/Elements/Series RLC Branch  LConnTagsString=__new0  RConnTagsString=__new0  BranchType=RL  Resistance=Rr  Inductance=Lr  SetiL0=off  InitialCurrent=0  Capacitance=10000e-6  Setx0=on  InitialVoltage=680  Measurements=None
  Series RLC Branch4 : powerlib/Elements/Series RLC Branch  LConnTagsString=__new0  RConnTagsString=__new0  BranchType=RL  Resistance=Rr  Inductance=Lr  SetiL0=off  InitialCurrent=0  Capacitance=10000e-6  Setx0=on  InitialVoltage=680  Measurements=None
  Series RLC Branch8 : powerlib/Elements/Series RLC Branch  LConnTagsString=__new0  RConnTagsString=__new0  BranchType=RL  Resistance=Rr  Inductance=Lr  SetiL0=off  InitialCurrent=0  Capacitance=10000e-6  Setx0=on  InitialVoltage=680  Measurements=None
  Series RLC Load2 : powerlib/Elements/Series RLC Load  LConnTagsString=a  RConnTagsString=__new0  NominalVoltage=48  NominalFrequency=60  ActivePower=3000  InductivePower=0  CapacitivePower=0  Setx0=off  InitialVoltage=0  SetiL0=off  InitialCurrent=0  Measurements=None  LoadType=constant Z
  Voltage Measurement1 : powerlib/Measurements/Voltage Measurement  PhasorSimulation=off  OutputType=Complex  PSBequivalent=0
  Voltage Measurement2 : powerlib/Measurements/Voltage Measurement  PhasorSimulation=off  OutputType=Complex  PSBequivalent=0
  Voltage Measurement3 : powerlib/Measurements/Voltage Measurement  PhasorSimulation=off  OutputType=Complex  PSBequivalent=0
  F1 : PMIOPort  Side=Left
  F2 : PMIOPort  Port=2  Side=Left
  F3 : PMIOPort  Port=3  Side=Left
  Van : Outport
  Vbn : Outport  Port=2
  Vcn : Outport  Port=3
  wires:
  Voltage Measurement1/1 -> Van/1
  Voltage Measurement2/1 -> Vbn/1
  Voltage Measurement3/1 -> Vcn/1
  connections:
  F1/RConn1 -- Series RLC Branch4/LConn1 -- Voltage Measurement1/LConn1
  F2/RConn1 -- Series RLC Branch3/LConn1 -- Voltage Measurement2/LConn1
  F3/RConn1 -- Series RLC Branch8/LConn1 -- Voltage Measurement3/LConn1
  Series RLC Branch3/RConn1 -- Series RLC Branch8/RConn1 -- Series RLC Branch4/RConn1 -- Voltage Measurement3/LConn2 -- Voltage Measurement2/LConn2 -- Voltage Measurement1/LConn2

== system MODELODETURBINADERIOV9/inversor/Controladores/Signal Builder ==
  Demux : Demux  Tag=STV Demux  Outputs=1
  FromWs : FromWorkspace  Tag=STV FromWs  VariableName=tuvar  SampleTime=0
      SigBuilderData=|
      | common.afterFinalStr = 'Extrapolate'
      | common.sampleTime = 0
      | dataSet.timeRange = [0 1]
      | dataSet.name = 'Group 1'
      | sbobj.Name = 'Signal Builder'
      | sbobj.Groups.Name = 'Group 1'
      | sbobj.Groups.Signals.Name = 'Signal 1'
      | sbobj.Groups.Signals.XData = [0 0.1 1]
      | sbobj.Groups.Signals.YData = [1 1 1]
      | sbobj.Groups.TimeRange = [0 1]
  Signal 1 : Outport  Tag=STV Outport
  wires:
  FromWs/1 -> Demux/1
  Demux/1 -> Signal 1/1

== matlab function MODELODETURBINADERIOV9/Turbina/MATLAB Function3 ==
  data: beta input; y output; landa input; Ii input
function y = fcn(beta, landa,Ii)
w=0.5176; 
w1=116/Ii;
 w2=0.4*beta;
 w3=exp(-21/Ii);
 
 cp=w*(w1-w2-5)*w3+0.0068*landa;
 
 
 
 
 
y=cp;

== matlab function MODELODETURBINADERIOV9/Turbina/Landai/lamdai ==
  data: beta input; Ii output; landa input
function Ii = fcn(beta,landa)


Iii=(1/((landa+(0.08*beta))))-((0.035)/((beta^3)+1));
Ii=1/Iii;
